simulink library "Pitch_TASK_Libs"  (Simulink 8.6)
settings: Solver=VariableStepAuto  SolverMode=SingleTasking  StartTime=0.0  StopTime=10.0  RelTol=1e-3
undefined symbols (not defined in the file or in its folder): M_SM_AUTO_RESET_TIME, M_SM_COUNTER_RESET_TIME
libraries: StandardLib x124, WindLib x7, Pitch_TASK_Libs x4, simulink x2
(part 1 of 2)
settings Model: Creator=300005582  LastModifiedBy=204050978

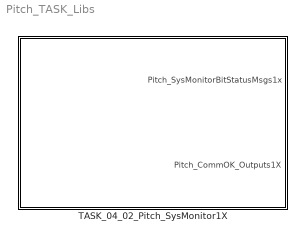
== system Pitch_TASK_Libs ==
  TASK_04_02_Pitch_SysMonitor1X : Subsystem  Priority=5
      settings: AttributesFormatString=ExecutionOrder = %<Priority>

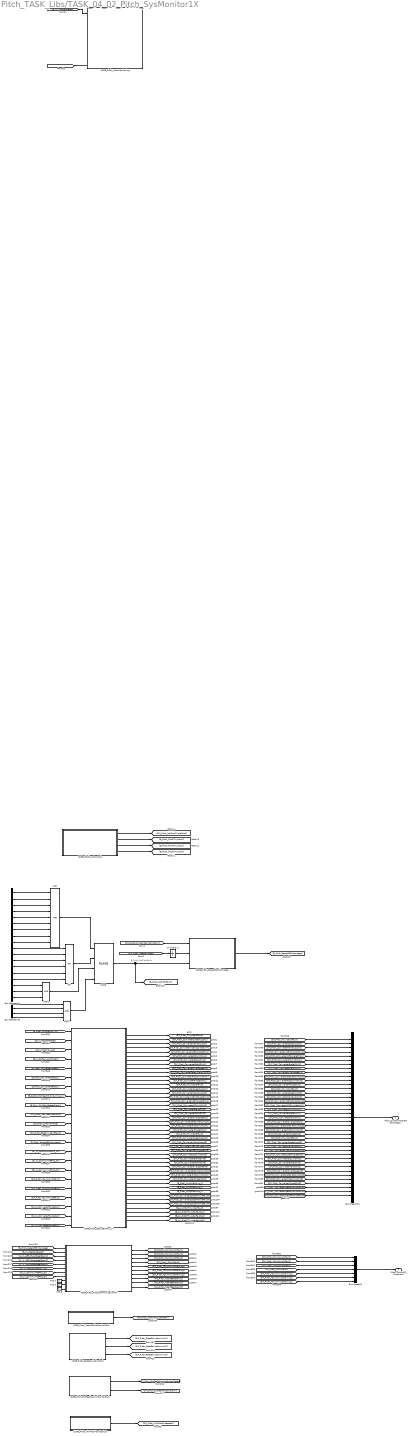
== system Pitch_TASK_Libs/TASK_04_02_Pitch_SysMonitor1X ==
  note: B_Pitch_NoPitchFault
  AND : StandardLib/Logical operations/AND  RepeatCnt=8  SampleTime=-1  ExecutionOrder=0
  AND1 : StandardLib/Logical operations/AND  RepeatCnt=3  SampleTime=-1  ExecutionOrder=0
  AND2 : StandardLib/Logical operations/AND  RepeatCnt=2  SampleTime=-1  ExecutionOrder=0
  Bus Creator10 : BusCreator  Inputs=39
  Bus Creator5 : BusCreator  Inputs=7  OutDataTypeStr=Bus: Pitch_CommOK_Outputs1X
  Bus Selector44 : BusSelector  OutputSignals=ExtInputs.DI_In_A1BattChargeOK,ExtInputs.DI_In_A2BattChargeOK,ExtInputs.DI_In_A3BattChargeOK,ExtInputs.DI_In_BattStringOKA1,ExtInputs.DI_In_BattStringOKA2,ExtInputs.DI_In_BattStringOKA3,ExtInputs.DI_In_BattVoltCompareOKA1,ExtInputs.DI_In_BattVoltCompareOKA2,ExtInputs.DI_In_BattVoltCompareOKA3,ExtInputs.DI_In_ConverterFaultedA1,ExtInputs.DI_In_ConverterFaultedA2,ExtInputs.DI_In_ConverterFaultedA3,ExtInputs.DI_In_MotorRTDFaultA1,ExtInputs.DI_In_MotorRTDFaultA2,ExtInputs.DI_In_MotorRTDFaultA3,ExtInputs.DI_In_CommunAEPA1_Ok,ExtInputs.DI_In_CommunAEPA2_Ok,ExtInputs.DI_In_CommunAEPA3_Ok
  Bus Selector45 : BusSelector  OutputSignals=Pitch_GlobalData.B_Pitch_Converter1Ready,Pitch_GlobalData.B_Pitch_Converter2Ready,Pitch_GlobalData.B_Pitch_Converter3Ready,OpCtl_GlobalData.B_OpCtl_PitchRectifyOnSummary
  OR : StandardLib/Logical operations/OR  RepeatCnt=5  SampleTime=-1  ExecutionOrder=0
  P13.1 : Constant  Value=0  OutDataTypeStr=boolean  SampleTime=-1
  P13.2 : Constant  Value=0  OutDataTypeStr=boolean  SampleTime=-1
  P13.3 : Constant  Value=0  OutDataTypeStr=boolean  SampleTime=-1
  RUNG : StandardLib/Logical operations/RUNG  Equation=A*(~B)*C*D  RepeatCount=4  SampleTime=-1  ExecutionOrder=0
  USRB_PitchSysMonStub : Subsystem  TreatAsAtomicUnit=on
      settings: MinAlgLoopOccurrences=on
  USRB_Pitch_ExtFeatherLimitSwitchStub : Subsystem  TreatAsAtomicUnit=on
  USRB_Pitch_MinPitchMonitorStub : Subsystem  TreatAsAtomicUnit=on
  USRB_Pitch_MotorCableMonitorStub : Subsystem  TreatAsAtomicUnit=on
  USRB_Pitch_MotorMonitoring : Subsystem  TreatAsAtomicUnit=on
  USRB_Pitch_PitchCommunicationOK : Subsystem  TreatAsAtomicUnit=on
  USRB_Pitch_RateDeviationStub : Subsystem  TreatAsAtomicUnit=on
  USRB_Pitch_ResetAftGridOutage : Subsystem  TreatAsAtomicUnit=on
  USRB_Pitch_StatusBitMon_1X : Subsystem  TreatAsAtomicUnit=on
  Unit Delay1 : UnitDelay  SampleTime=-1
  Pitch_SysMonitorBitStatusMsgs1x : Outport  OutDataTypeStr=Bus: Pitch_SysMonitor_LocalData1X
  Pitch_CommOK_Outputs1X : Outport  Port=2  OutDataTypeStr=Bus: Pitch_CommOK_Outputs1X
  wires:
  USRB_PitchSysMonStub/4(B_Pitch_PitchThysitor3) -> [B_Pitch_PitchThysitor3]  "B_Pitch_PitchThysitor3"
  USRB_PitchSysMonStub/2(B_Pitch_PitchThysitor1) -> [B_Pitch_PitchThysitor1]  "B_Pitch_PitchThysitor1"
  USRB_PitchSysMonStub/3(B_Pitch_PitchThysitor2) -> [B_Pitch_PitchThysitor2]  "B_Pitch_PitchThysitor2"
  USRB_PitchSysMonStub/1(SM_Pitch_MalfuncTriplePitch) -> [SM_Pitch_MalfuncTriplePitch]  "SM_Pitch_MalfuncTriplePitch"
  OR/1 -> RUNG/2
  AND/1 -> RUNG/1
  [SM_OpCtl_SystemReinitalization] -> USRB_Pitch_ResetAftGridOutage/1(SM_OpCtl_SystemReinitalization)
  USRB_Pitch_ResetAftGridOutage/1(B_Pitch_ResetAftGridoutage) -> [B_Pitch_ResetAftGridoutage]  "B_Pitch_ResetAftGridouate"
  Bus Selector44/1 -> AND/1  "<DI_In_A1BattChargeOK>"
  Bus Selector44/2 -> AND/2  "<DI_In_A2BattChargeOK>"
  Bus Selector44/3 -> AND/3  "<DI_In_A3BattChargeOK>"
  Bus Selector44/4 -> AND/4  "<DI_In_BattStringOKA1>"
  Bus Selector44/5 -> AND/5  "<DI_In_BattStringOKA2>"
  Bus Selector44/6 -> AND/6  "<DI_In_BattStringOKA3>"
  Bus Selector44/7 -> AND/7  "<DI_In_BattVoltCompareOKA1>"
  Bus Selector44/8 -> AND/8  "<DI_In_BattVoltCompareOKA2>"
  Bus Selector44/9 -> AND/9  "<DI_In_BattVoltCompareOKA3>"
  Bus Selector44/10 -> OR/1  "<DI_In_ConverterFaultedA1>"
  Bus Selector44/11 -> OR/2  "<DI_In_ConverterFaultedA2>"
  Bus Selector44/12 -> OR/3  "<DI_In_ConverterFaultedA3>"
  Bus Selector44/13 -> OR/4  "<DI_In_MotorRTDFaultA1>"
  Bus Selector44/14 -> OR/5  "<DI_In_MotorRTDFaultA2>"
  Bus Selector44/15 -> OR/6  "<DI_In_MotorRTDFaultA3>"
  RUNG/1 -> USRB_Pitch_ResetAftGridOutage/3(Pich_GeneralOK), [B_Pitch_NoPitchFault]
  Bus Selector45/1 -> AND1/1  "<B_Pitch_Converter1Ready>"
  Bus Selector45/2 -> AND1/2  "<B_Pitch_Converter2Ready>"
  Bus Selector45/3 -> AND1/3  "<B_Pitch_Converter3Ready>"
  Bus Selector45/4 -> AND1/4  "<B_OpCtl_PitchRectifyOnSummary>"
  Bus Selector44/16 -> AND2/1  "<DI_In_CommunAEPA1_Ok>"
  Bus Selector44/17 -> AND2/2  "<DI_In_CommunAEPA2_Ok>"
  Bus Selector44/18 -> AND2/3  "<DI_In_CommunAEPA3_Ok>"
  AND1/1 -> RUNG/4
  AND2/1 -> RUNG/3
  [SM_Pitch_InternalMode] -> Unit Delay1/1
  Unit Delay1/1 -> USRB_Pitch_ResetAftGridOutage/2(SM_Pitch_InternalMode)
  [B_Pitch_ResetAftGridoutage] -> ?
  [B_In_WtgStartReset] -> USRB_Pitch_MotorMonitoring/1(B_In_WtgStartReset)
  USRB_Pitch_StatusBitMon_1X/1(SM_Pitch_Thyristor1Fault) -> [SM_Pitch_Thyristor1Fault]  "SM_Pitch_Thyristor1Fault"
  USRB_Pitch_StatusBitMon_1X/2(SM_Pitch_ConverterSpeedLossA1) -> [SM_Pitch_ConverterSpeedLossA1]  "SM_Pitch_ConverterSpeedLossA1"
  USRB_Pitch_StatusBitMon_1X/3(SM_Pitch_ConverterMarkerLossA1) -> [SM_Pitch_ConverterMarkerLossA1]  "SM_Pitch_ConverterMarkerLossA1"
  USRB_Pitch_StatusBitMon_1X/4(SM_Pitch_ConverterIncEncCorrectionA1) -> [SM_Pitch_ConverterIncEncCorrectionA1]  "SM_Pitch_ConverterIncEncCorrectionA1"
  USRB_Pitch_StatusBitMon_1X/5(SM_Pitch_ConverterLS90AngleErrA1) -> [SM_Pitch_ConverterLS90AngleErrA1]  "SM_Pitch_ConverterLS90AngleErrA1"
  USRB_Pitch_StatusBitMon_1X/6(SM_Pitch_ConverterDCLinkOKA1) -> [SM_Pitch_ConverterDCLinkOKA1]  "SM_Pitch_ConverterDCLinkOKA1"
  USRB_Pitch_StatusBitMon_1X/7(SM_Pitch_ConverterBrakeOKA1) -> [SM_Pitch_ConverterBrakeOKA1]  "SM_Pitch_ConverterBrakeOKA1"
  USRB_Pitch_StatusBitMon_1X/8(SM_Pitch_ConverterFieldOKA1) -> [SM_Pitch_ConverterFieldOKA1]  "SM_Pitch_ConverterFieldOKA1"
  USRB_Pitch_StatusBitMon_1X/9(SM_Pitch_ConverterOverSpeedA1) -> [SM_Pitch_ConverterOverSpeedA1]  "SM_Pitch_ConverterOverSpeedA1"
  USRB_Pitch_StatusBitMon_1X/10(SM_Pitch_ConverterSafetyRelayPLCA1) -> [SM_Pitch_ConverterSafetyRelayPLCA1]  "SM_Pitch_ConverterSafetyRelayPLCA1"
  USRB_Pitch_StatusBitMon_1X/11(SM_Pitch_ConverterPICCommOKA1) -> [SM_Pitch_ConverterPICCommOKA1]  "SM_Pitch_ConverterPICCommOKA1"
  USRB_Pitch_StatusBitMon_1X/12(SM_Pitch_ConverterPhaseOkA1) -> [SM_Pitch_ConverterPhaseOkA1]  "SM_Pitch_ConverterPhaseOkA1"
  USRB_Pitch_StatusBitMon_1X/13(SM_Pitch_Thyristor2Fault) -> [SM_Pitch_Thyristor2Fault]  "SM_Pitch_Thyristor2Fault"
  USRB_Pitch_StatusBitMon_1X/14(SM_Pitch_ConverterSpeedLossA2) -> [SM_Pitch_ConverterSpeedLossA2]  "SM_Pitch_ConverterSpeedLossA2"
  USRB_Pitch_StatusBitMon_1X/15(SM_Pitch_ConverterMarkerLossA2) -> [SM_Pitch_ConverterMarkerLossA2]  "SM_Pitch_ConverterMarkerLossA2"
  USRB_Pitch_StatusBitMon_1X/16(SM_Pitch_ConverterIncEncCorrectionA2) -> [SM_Pitch_ConverterIncEncCorrectionA2]  "SM_Pitch_ConverterIncEncCorrectionA2"
  USRB_Pitch_StatusBitMon_1X/17(SM_Pitch_ConverterLS90AngleErrA2) -> [SM_Pitch_ConverterLS90AngleErrA2]  "SM_Pitch_ConverterLS90AngleErrA2"
  USRB_Pitch_StatusBitMon_1X/18(SM_Pitch_ConverterDCLinkOKA2) -> [SM_Pitch_ConverterDCLinkOKA2]  "SM_Pitch_ConverterDCLinkOKA2"
  USRB_Pitch_StatusBitMon_1X/19(SM_Pitch_ConverterBrakeOKA2) -> [SM_Pitch_ConverterBrakeOKA2]  "SM_Pitch_ConverterBrakeOKA2"
  USRB_Pitch_StatusBitMon_1X/20(SM_Pitch_ConverterFieldOKA2) -> [SM_Pitch_ConverterFieldOKA2]  "SM_Pitch_ConverterFieldOKA2"
  USRB_Pitch_StatusBitMon_1X/21(SM_Pitch_ConverterOverSpeedA2) -> [SM_Pitch_ConverterOverSpeedA2]  "SM_Pitch_ConverterOverSpeedA2"
  USRB_Pitch_StatusBitMon_1X/22(SM_Pitch_ConverterSafetyRelayPLCA2) -> [SM_Pitch_ConverterSafetyRelayPLCA2]  "SM_Pitch_ConverterSafetyRelayPLCA2"
  USRB_Pitch_StatusBitMon_1X/23(SM_Pitch_ConverterPICCommOKA2) -> [SM_Pitch_ConverterPICCommOKA2]  "SM_Pitch_ConverterPICCommOKA2"
  USRB_Pitch_StatusBitMon_1X/24(SM_Pitch_ConverterPhaseOkA2) -> [SM_Pitch_ConverterPhaseOkA2]  "SM_Pitch_ConverterPhaseOkA2"
  USRB_Pitch_StatusBitMon_1X/25(SM_Pitch_Thyristor3Fault) -> [SM_Pitch_Thyristor3Fault]  "SM_Pitch_Thyristor3Fault"
  USRB_Pitch_StatusBitMon_1X/26(SM_Pitch_ConverterSpeedLossA3) -> [SM_Pitch_ConverterSpeedLossA3]  "SM_Pitch_ConverterSpeedLossA3"
  USRB_Pitch_StatusBitMon_1X/27(SM_Pitch_ConverterMarkerLossA3) -> [SM_Pitch_ConverterMarkerLossA3]  "SM_Pitch_ConverterMarkerLossA3"
  USRB_Pitch_StatusBitMon_1X/28(SM_Pitch_ConverterIncEncCorrectionA3) -> [SM_Pitch_ConverterIncEncCorrectionA3]  "SM_Pitch_ConverterIncEncCorrectionA3"
  USRB_Pitch_StatusBitMon_1X/29(SM_Pitch_ConverterLS90AngleErrA3) -> [SM_Pitch_ConverterLS90AngleErrA3]  "SM_Pitch_ConverterLS90AngleErrA3"
  USRB_Pitch_StatusBitMon_1X/30(SM_Pitch_ConverterDCLinkOKA3) -> [SM_Pitch_ConverterDCLinkOKA3]  "SM_Pitch_ConverterDCLinkOKA3"
  USRB_Pitch_StatusBitMon_1X/31(SM_Pitch_ConverterBrakeOKA3) -> [SM_Pitch_ConverterBrakeOKA3]  "SM_Pitch_ConverterBrakeOKA3"
  USRB_Pitch_StatusBitMon_1X/32(SM_Pitch_ConverterFieldOKA3) -> [SM_Pitch_ConverterFieldOKA3]  "SM_Pitch_ConverterFieldOKA3"
  USRB_Pitch_StatusBitMon_1X/33(SM_Pitch_ConverterOverSpeedA3) -> [SM_Pitch_ConverterOverSpeedA3]  "SM_Pitch_ConverterOverSpeedA3"
  USRB_Pitch_StatusBitMon_1X/34(SM_Pitch_ConverterSafetyRelayPLCA3) -> [SM_Pitch_ConverterSafetyRelayPLCA3]  "SM_Pitch_ConverterSafetyRelayPLCA3"
  USRB_Pitch_StatusBitMon_1X/35(SM_Pitch_ConverterPICCommOKA3) -> [SM_Pitch_ConverterPICCommOKA3]  "SM_Pitch_ConverterPICCommOKA3"
  USRB_Pitch_StatusBitMon_1X/36(SM_Pitch_ConverterPhaseOkA3) -> [SM_Pitch_ConverterPhaseOkA3]  "SM_Pitch_ConverterPhaseOkA3"
  USRB_Pitch_StatusBitMon_1X/37(B_Pitch_Axis1Malfunc_L) -> [B_Pitch_Axis1Malfunc_L]
  USRB_Pitch_StatusBitMon_1X/38(B_Pitch_Axis2Malfunc_L) -> [B_Pitch_Axis2Malfunc_L]
  USRB_Pitch_StatusBitMon_1X/39(B_Pitch_Axis3Malfunc_L) -> [B_Pitch_Axis3Malfunc_L]
  [B_Pitch_AxisMalFun_LL] -> USRB_Pitch_StatusBitMon_1X/1(B_Pitch_AxisMalFun_LL)
  [B_In_WtgStartReset] -> USRB_Pitch_StatusBitMon_1X/2(B_In_WtgStartReset)
  [C_In_PitchManual] -> USRB_Pitch_StatusBitMon_1X/3(C_In_PitchManual)
  [B_In_SafetyLoopClosed] -> USRB_Pitch_StatusBitMon_1X/4(B_In_SafetyLoopClosed)
  [B_Pitch_Converter1Ready] -> USRB_Pitch_StatusBitMon_1X/5(B_Pitch_Converter1Ready)
  [B_Pitch_Converter2Ready] -> USRB_Pitch_StatusBitMon_1X/6(B_Pitch_Converter2Ready)
  [B_Pitch_Converter3Ready] -> USRB_Pitch_StatusBitMon_1X/7(B_Pitch_Converter3Ready)
  [B_OpCtl_PitchRectifyOnSummary] -> USRB_Pitch_StatusBitMon_1X/8(B_OpCtl_PitchRectifyOnSummary)
  [B_Envr_GridFaultResetDelay] -> USRB_Pitch_StatusBitMon_1X/9(B_Envr_GridFaultResetDelay)
  [SM_Pitch_ServiceSwitchHub] -> USRB_Pitch_StatusBitMon_1X/10(SM_Pitch_ServiceSwitchHub)
  [SM_Pitch_InternalMode] -> USRB_Pitch_StatusBitMon_1X/11(SM_Pitch_InternalMode)
  [SM_Pitch_BattDriveGridFault] -> USRB_Pitch_StatusBitMon_1X/12(SM_Pitch_BattDriveGridFault)
  [B_Pitch_ResetAftGridoutage] -> USRB_Pitch_StatusBitMon_1X/13(B_Pitch_ResetAftGridoutage)
  [DI_In_CommunAEPA1_Ok] -> USRB_Pitch_StatusBitMon_1X/14(DI_In_CommunAEPA1_Ok)
  [DI_In_CommunAEPA2_Ok] -> USRB_Pitch_StatusBitMon_1X/15(DI_In_CommunAEPA2_Ok)
  [DI_In_CommunAEPA3_Ok] -> USRB_Pitch_StatusBitMon_1X/16(DI_In_CommunAEPA3_Ok)
  [SM_Pitch_IOLinkAxis1Fault] -> USRB_Pitch_StatusBitMon_1X/17(SM_Pitch_IOLinkAxis1Fault)
  [SM_Pitch_IOLinkAxis2Fault] -> USRB_Pitch_StatusBitMon_1X/18(SM_Pitch_IOLinkAxis2Fault)
  [SM_Pitch_IOLinkAxis3Fault] -> USRB_Pitch_StatusBitMon_1X/19(SM_Pitch_IOLinkAxis3Fault)
  [DI_In_ConverterFaultedA1] -> USRB_Pitch_StatusBitMon_1X/20(DI_In_ConverterFaultedA1)
  [DI_In_ConverterFaultedA2] -> USRB_Pitch_StatusBitMon_1X/21(DI_In_ConverterFaultedA2)
  [DI_In_ConverterFaultedA3] -> USRB_Pitch_StatusBitMon_1X/22(DI_In_ConverterFaultedA3)
  USRB_Pitch_StatusBitMon_1X/43(B_AnyPitchThyristorFault) -> [B_AnyPitchThyristorFault]
  USRB_Pitch_PitchCommunicationOK/1(SM_Pitch_IOLinkAxis1Fault) -> [SM_Pitch_IOLinkAxis1Fault]
  USRB_Pitch_PitchCommunicationOK/2(SM_Pitch_IOLinkAxis2Fault) -> [SM_Pitch_IOLinkAxis2Fault]
  USRB_Pitch_PitchCommunicationOK/3(SM_Pitch_IOLinkAxis3Fault) -> [SM_Pitch_IOLinkAxis3Fault]
  USRB_Pitch_PitchCommunicationOK/4(SM_Pitch_IOLinkFault) -> [SM_Pitch_IOLinkFault]
  USRB_Pitch_PitchCommunicationOK/5(SM_Pitch_IOLinkAxis1Warning) -> [SM_Pitch_IOLinkAxis1Warning]
  USRB_Pitch_PitchCommunicationOK/6(SM_Pitch_IOLinkAxis2Warning) -> [SM_Pitch_IOLinkAxis2Warning]
  USRB_Pitch_PitchCommunicationOK/7(SM_Pitch_IOLinkAxis3Warning) -> [SM_Pitch_IOLinkAxis3Warning]
  USRB_Pitch_PitchCommunicationOK/8(AO_Pitch_HeartBeatSend1) -> [AO_Pitch_HeartBeatSend1]
  USRB_Pitch_PitchCommunicationOK/9(AO_Pitch_HeartBeatSend2) -> [AO_Pitch_HeartBeatSend2]
  USRB_Pitch_PitchCommunicationOK/10(AO_Pitch_HeartBeatSend3) -> [AO_Pitch_HeartBeatSend3]
  [B_Pitch_ResetAftGridoutage] -> USRB_Pitch_PitchCommunicationOK/1(B_Pitch_ResetAftGridoutage)
  [B_In_WtgStartReset] -> USRB_Pitch_PitchCommunicationOK/2(B_In_WtgStartReset)
  [AI_In_AEPAHeartbeatRecv1] -> USRB_Pitch_PitchCommunicationOK/3(AI_In_AEPAHeartbeatRecv1)
  [AI_In_AEPAHeartbeatRecv2] -> USRB_Pitch_PitchCommunicationOK/4(AI_In_AEPAHeartbeatRecv2)
  [AI_In_AEPAHeartbeatRecv3] -> USRB_Pitch_PitchCommunicationOK/5(AI_In_AEPAHeartbeatRecv3)
  [DI_In_CommunAEPA1_Ok] -> USRB_Pitch_PitchCommunicationOK/6(DI_In_CommunAEPA1_Ok)
  [DI_In_CommunAEPA2_Ok] -> USRB_Pitch_PitchCommunicationOK/7(DI_In_CommunAEPA2_Ok)
  [DI_In_CommunAEPA3_Ok] -> USRB_Pitch_PitchCommunicationOK/8(DI_In_CommunAEPA3_Ok)
  P13.1/1 -> USRB_Pitch_PitchCommunicationOK/9(B_TestShortTimeComFault)
  P13.2/1 -> USRB_Pitch_PitchCommunicationOK/10(B_TestLongTimeComFaultTwoAxes)
  P13.3/1 -> USRB_Pitch_PitchCommunicationOK/11(B_TestLongTimeComFaultAllAxes)
  Bus Creator10/1 -> Pitch_SysMonitorBitStatusMsgs1x/1  "Pitch_SysMonitorBitStatusMsgs1x"
  [SM_Pitch_Thyristor1Fault] -> Bus Creator10/1  "SM_Pitch_Thyristor1Fault"
  [SM_Pitch_ConverterSpeedLossA1] -> Bus Creator10/2  "SM_Pitch_ConverterSpeedLossA1"
  [SM_Pitch_ConverterMarkerLossA1] -> Bus Creator10/3  "SM_Pitch_ConverterMarkerLossA1"
  [SM_Pitch_ConverterIncEncCorrectionA1] -> Bus Creator10/4  "SM_Pitch_ConverterIncEncCorrectionA1"
  [SM_Pitch_ConverterLS90AngleErrA1] -> Bus Creator10/5  "SM_Pitch_ConverterLS90AngleErrA1"
  [SM_Pitch_ConverterDCLinkOKA1] -> Bus Creator10/6  "SM_Pitch_ConverterDCLinkOKA1"
  [SM_Pitch_ConverterBrakeOKA1] -> Bus Creator10/7  "SM_Pitch_ConverterBrakeOKA1"
  [SM_Pitch_ConverterFieldOKA1] -> Bus Creator10/8  "SM_Pitch_ConverterFieldOKA1"
  [SM_Pitch_ConverterOverSpeedA1] -> Bus Creator10/9  "SM_Pitch_ConverterOverSpeedA1"
  [SM_Pitch_ConverterSafetyRelayPLCA1] -> Bus Creator10/10  "SM_Pitch_ConverterSafetyRelayPLCA1"
  [SM_Pitch_ConverterPICCommOKA1] -> Bus Creator10/11  "SM_Pitch_ConverterPICCommOKA1"
  [SM_Pitch_ConverterPhaseOkA1] -> Bus Creator10/12  "SM_Pitch_ConverterPhaseOkA1"
  [SM_Pitch_Thyristor2Fault] -> Bus Creator10/13  "SM_Pitch_Thyristor2Fault"
  [SM_Pitch_ConverterSpeedLossA2] -> Bus Creator10/14  "SM_Pitch_ConverterSpeedLossA2"
  [SM_Pitch_ConverterMarkerLossA2] -> Bus Creator10/15  "SM_Pitch_ConverterMarkerLossA2"
  [SM_Pitch_ConverterIncEncCorrectionA2] -> Bus Creator10/16  "SM_Pitch_ConverterIncEncCorrectionA2"
  [SM_Pitch_ConverterLS90AngleErrA2] -> Bus Creator10/17  "SM_Pitch_ConverterLS90AngleErrA2"
  [SM_Pitch_ConverterDCLinkOKA2] -> Bus Creator10/18  "SM_Pitch_ConverterDCLinkOKA2"
  [SM_Pitch_ConverterBrakeOKA2] -> Bus Creator10/19  "SM_Pitch_ConverterBrakeOKA2"
  [SM_Pitch_ConverterFieldOKA2] -> Bus Creator10/20  "SM_Pitch_ConverterFieldOKA2"
  [SM_Pitch_ConverterOverSpeedA2] -> Bus Creator10/21  "SM_Pitch_ConverterOverSpeedA2"
  [SM_Pitch_ConverterSafetyRelayPLCA2] -> Bus Creator10/22  "SM_Pitch_ConverterSafetyRelayPLCA2"
  [SM_Pitch_ConverterPICCommOKA2] -> Bus Creator10/23  "SM_Pitch_ConverterPICCommOKA2"
  [SM_Pitch_ConverterPhaseOkA2] -> Bus Creator10/24  "SM_Pitch_ConverterPhaseOkA2"
  [SM_Pitch_Thyristor3Fault] -> Bus Creator10/25  "SM_Pitch_Thyristor3Fault"
  [SM_Pitch_ConverterSpeedLossA3] -> Bus Creator10/26  "SM_Pitch_ConverterSpeedLossA3"
  [SM_Pitch_ConverterMarkerLossA3] -> Bus Creator10/27  "SM_Pitch_ConverterMarkerLossA3"
  [SM_Pitch_ConverterIncEncCorrectionA3] -> Bus Creator10/28  "SM_Pitch_ConverterIncEncCorrectionA3"
  [SM_Pitch_ConverterLS90AngleErrA3] -> Bus Creator10/29  "SM_Pitch_ConverterLS90AngleErrA3"
  [SM_Pitch_ConverterDCLinkOKA3] -> Bus Creator10/30  "SM_Pitch_ConverterDCLinkOKA3"
  [SM_Pitch_ConverterBrakeOKA3] -> Bus Creator10/31  "SM_Pitch_ConverterBrakeOKA3"
  [SM_Pitch_ConverterFieldOKA3] -> Bus Creator10/32  "SM_Pitch_ConverterFieldOKA3"
  [SM_Pitch_ConverterOverSpeedA3] -> Bus Creator10/33  "SM_Pitch_ConverterOverSpeedA3"
  [SM_Pitch_ConverterSafetyRelayPLCA3] -> Bus Creator10/34  "SM_Pitch_ConverterSafetyRelayPLCA3"
  [SM_Pitch_ConverterPICCommOKA3] -> Bus Creator10/35  "SM_Pitch_ConverterPICCommOKA3"
  [SM_Pitch_ConverterPhaseOkA3] -> Bus Creator10/36  "SM_Pitch_ConverterPhaseOkA3"
  USRB_Pitch_StatusBitMon_1X/40(SM_Pitch_ConverterSpeedProfileFaultA1) -> [SM_Pitch_ConverterSpeedProfileFaultA1]
  USRB_Pitch_StatusBitMon_1X/41(SM_Pitch_ConverterSpeedProfileFaultA2) -> [SM_Pitch_ConverterSpeedProfileFaultA2]
  USRB_Pitch_StatusBitMon_1X/42(SM_Pitch_ConverterSpeedProfileFaultA3) -> [SM_Pitch_ConverterSpeedProfileFaultA3]
  [SM_Pitch_ConverterSpeedProfileFaultA1] -> Bus Creator10/37  "SM_Pitch_ConverterSpeedProfileFaultA1"
  [SM_Pitch_ConverterSpeedProfileFaultA2] -> Bus Creator10/38  "SM_Pitch_ConverterSpeedProfileFaultA2"
  [SM_Pitch_ConverterSpeedProfileFaultA3] -> Bus Creator10/39  "SM_Pitch_ConverterSpeedProfileFaultA3"
  USRB_Pitch_StatusBitMon_1X/44(B_AnyPitchThyristorFaultA1) -> [B_AnyPitchThyristorFaultA1]
  USRB_Pitch_StatusBitMon_1X/45(B_AnyPitchThyristorFaultA2) -> [B_AnyPitchThyristorFaultA2]
  USRB_Pitch_StatusBitMon_1X/46(B_AnyPitchThyristorFaultA3) -> [B_AnyPitchThyristorFaultA3]
  USRB_Pitch_MotorCableMonitorStub/1(SM_Pitch_PitchMotorCableFail) -> [SM_Pitch_PitchMotorCableFail]
  USRB_Pitch_RateDeviationStub/1(SM_Pitch_RateDeviationAxis1) -> [SM_Pitch_RateDeviationAxis1]
  USRB_Pitch_RateDeviationStub/2(SM_Pitch_RateDeviationAxis2) -> [SM_Pitch_RateDeviationAxis2]
  USRB_Pitch_RateDeviationStub/3(SM_Pitch_RateDeviationAxis3) -> [SM_Pitch_RateDeviationAxis3]
  USRB_Pitch_ExtFeatherLimitSwitchStub/1(SM_Pitch_ExtFeathPosLmtSwitchDefect) -> [SM_Pitch_ExtFeathPosLmtSwitchDefect]
  USRB_Pitch_ExtFeatherLimitSwitchStub/2(SM_Pitch_ExtFeathPosOverRun) -> [SM_Pitch_ExtFeathPosOverRun]
  USRB_Pitch_MinPitchMonitorStub/1(SM_Pitch_MinPitchExceeded) -> [SM_Pitch_MinPitchExceeded]
  [SM_Pitch_IOLinkAxis1Fault] -> Bus Creator5/1  "SM_Pitch_IOLinkAxis1Fault"
  [SM_Pitch_IOLinkAxis2Fault] -> Bus Creator5/2  "SM_Pitch_IOLinkAxis2Fault"
  [SM_Pitch_IOLinkAxis3Fault] -> Bus Creator5/3  "SM_Pitch_IOLinkAxis3Fault"
  [SM_Pitch_IOLinkFault] -> Bus Creator5/4  "SM_Pitch_IOLinkFault"
  [SM_Pitch_IOLinkAxis1Warning] -> Bus Creator5/5  "SM_Pitch_IOLinkAxis1Warning"
  [SM_Pitch_IOLinkAxis2Warning] -> Bus Creator5/6  "SM_Pitch_IOLinkAxis2Warning"
  [SM_Pitch_IOLinkAxis3Warning] -> Bus Creator5/7  "SM_Pitch_IOLinkAxis3Warning"
  Bus Creator5/1 -> Pitch_CommOK_Outputs1X/1  "Pitch_CommOK_Outputs1X"

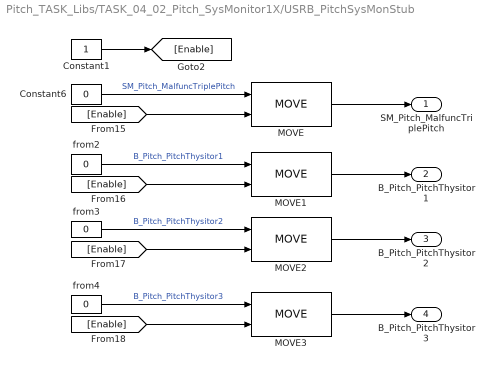
== system Pitch_TASK_Libs/TASK_04_02_Pitch_SysMonitor1X/USRB_PitchSysMonStub ==
  Constant1 : Constant  OutDataTypeStr=boolean
  Constant6 : Constant  Value=0  OutDataTypeStr=boolean
  MOVE{,1..3} (4 alike) : StandardLib/Memory operations/MOVE  DataType=BOOLEAN  SampleTime=-1  ExecutionOrder=0
  from2 : Constant  Value=0  OutDataTypeStr=boolean
  from3 : Constant  Value=0  OutDataTypeStr=boolean
  from4 : Constant  Value=0  OutDataTypeStr=boolean
  SM_Pitch_MalfuncTriplePitch : Outport  OutDataTypeStr=boolean
  B_Pitch_PitchThysitor1 : Outport  Port=2  OutDataTypeStr=boolean
  B_Pitch_PitchThysitor2 : Outport  Port=3  OutDataTypeStr=boolean
  B_Pitch_PitchThysitor3 : Outport  Port=4  OutDataTypeStr=boolean
  wires:
  from2/1 -> MOVE1/1  "B_Pitch_PitchThysitor1"
  from3/1 -> MOVE2/1  "B_Pitch_PitchThysitor2"
  from4/1 -> MOVE3/1  "B_Pitch_PitchThysitor3"
  Constant6/1 -> MOVE/1  "SM_Pitch_MalfuncTriplePitch"
  [Enable] -> MOVE/2
  [Enable] -> MOVE1/2
  [Enable] -> MOVE2/2
  [Enable] -> MOVE3/2
  MOVE/1 -> SM_Pitch_MalfuncTriplePitch/1
  MOVE1/1 -> B_Pitch_PitchThysitor1/1
  MOVE2/1 -> B_Pitch_PitchThysitor2/1
  MOVE3/1 -> B_Pitch_PitchThysitor3/1
  Constant1/1 -> [Enable]

== system Pitch_TASK_Libs/TASK_04_02_Pitch_SysMonitor1X/USRB_Pitch_ExtFeatherLimitSwitchStub ==
  Constant1 : Constant  Value=0  OutDataTypeStr=boolean
  Constant18 : Constant  Value=0  OutDataTypeStr=boolean
  Constant19 : Constant  OutDataTypeStr=boolean
  Constant2 : Constant  OutDataTypeStr=boolean
  MOVE1 : StandardLib/Memory operations/MOVE  DataType=BOOLEAN  SampleTime=-1  ExecutionOrder=0
  MOVE9 : StandardLib/Memory operations/MOVE  DataType=BOOLEAN  SampleTime=-1  ExecutionOrder=0
  SM_Pitch_ExtFeathPosLmtSwitchDefect : Outport  OutDataTypeStr=boolean
  SM_Pitch_ExtFeathPosOverRun : Outport  Port=2  OutDataTypeStr=boolean
  wires:
  Constant19/1 -> MOVE9/2
  Constant18/1 -> MOVE9/1
  MOVE9/1 -> SM_Pitch_ExtFeathPosLmtSwitchDefect/1
  Constant2/1 -> MOVE1/2
  Constant1/1 -> MOVE1/1
  MOVE1/1 -> SM_Pitch_ExtFeathPosOverRun/1

== system Pitch_TASK_Libs/TASK_04_02_Pitch_SysMonitor1X/USRB_Pitch_MinPitchMonitorStub ==
  note: ***********************************************************************************************************************************************
      | ***********         Change history. Please include your changes below and in the in the modified Task / USRB         ***********
      | ***********************************************************************************************************************************************
      | 2013-01-11, JGC: Corrected logic of SM450. SUB block substituted by ADD block in threshold calculation
      | 2013-07-25, JGC: SM450 is masked during 5s after LVRT
  Constant18 : Constant  Value=0  OutDataTypeStr=boolean
  Constant19 : Constant  OutDataTypeStr=boolean
  MOVE9 : StandardLib/Memory operations/MOVE  DataType=BOOLEAN  SampleTime=-1  ExecutionOrder=0
  SM_Pitch_MinPitchExceeded : Outport  OutDataTypeStr=boolean
  wires:
  Constant19/1 -> MOVE9/2
  Constant18/1 -> MOVE9/1
  MOVE9/1 -> SM_Pitch_MinPitchExceeded/1

== system Pitch_TASK_Libs/TASK_04_02_Pitch_SysMonitor1X/USRB_Pitch_MotorCableMonitorStub ==
  Constant18 : Constant  Value=0  OutDataTypeStr=boolean
  Constant19 : Constant  OutDataTypeStr=boolean
  MOVE9 : StandardLib/Memory operations/MOVE  DataType=BOOLEAN  SampleTime=-1  ExecutionOrder=0
  SM_Pitch_PitchMotorCableFail : Outport  OutDataTypeStr=boolean
  wires:
  Constant19/1 -> MOVE9/2
  Constant18/1 -> MOVE9/1
  MOVE9/1 -> SM_Pitch_PitchMotorCableFail/1

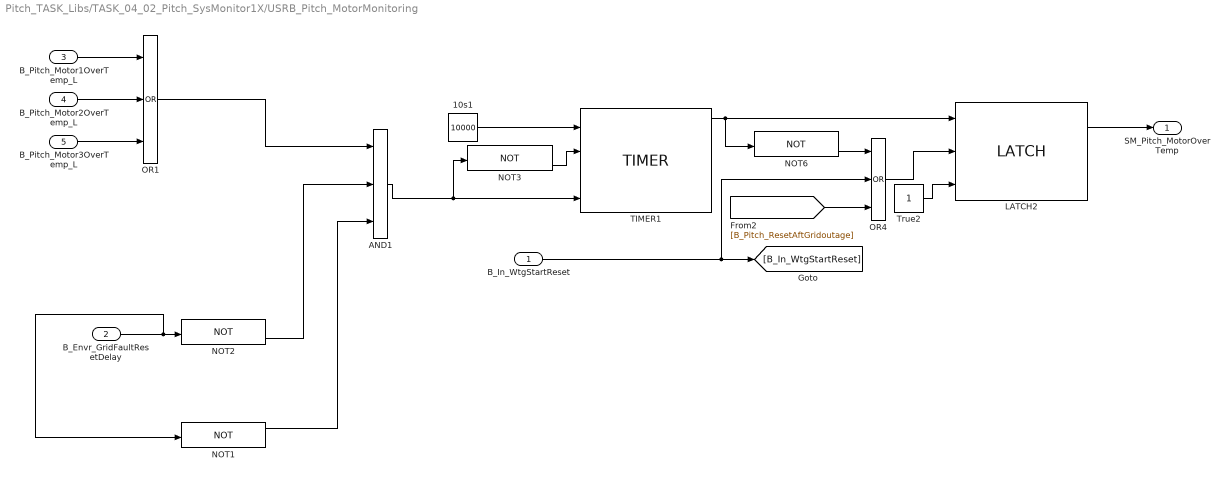
== system Pitch_TASK_Libs/TASK_04_02_Pitch_SysMonitor1X/USRB_Pitch_MotorMonitoring ==
  B_In_WtgStartReset : Inport  OutDataTypeStr=boolean
  B_Envr_GridFaultResetDelay : Inport  Port=2  OutDataTypeStr=boolean
  B_Pitch_Motor1OverTemp_L : Inport  Port=3  OutDataTypeStr=boolean
  B_Pitch_Motor2OverTemp_L : Inport  Port=4  OutDataTypeStr=boolean
  B_Pitch_Motor3OverTemp_L : Inport  Port=5  OutDataTypeStr=boolean
  10s1 : Constant  Value=10000  OutDataTypeStr=uint32  SampleTime=-1
  AND1 : StandardLib/Logical operations/AND  RepeatCnt=2  SampleTime=-1  ExecutionOrder=0
  LATCH2 : StandardLib/Logical operations/LATCH  SampleTime=-1  ExecutionOrder=0
  NOT{1..3,6} (4 alike) : StandardLib/Logical operations/NOT  SampleTime=-1  ExecutionOrder=0
  OR1 : StandardLib/Logical operations/OR  RepeatCnt=2  SampleTime=-1  ExecutionOrder=0
  OR4 : StandardLib/Logical operations/OR  RepeatCnt=2  SampleTime=-1  ExecutionOrder=0
  TIMER1 : StandardLib/Timers and Counters/TIMER  SampleTime=-1  ExecutionOrder=0
  True2 : Constant  OutDataTypeStr=boolean  SampleTime=-1
  SM_Pitch_MotorOverTemp : Outport  OutDataTypeStr=boolean
  wires:
  NOT6/2 -> OR4/1
  TIMER1/1 -> LATCH2/1, NOT6/1
  B_In_WtgStartReset/1 -> [B_In_WtgStartReset], OR4/2
  B_Pitch_Motor3OverTemp_L/1 -> OR1/3
  B_Pitch_Motor2OverTemp_L/1 -> OR1/2
  B_Pitch_Motor1OverTemp_L/1 -> OR1/1
  NOT3/2 -> TIMER1/2
  10s1/1 -> TIMER1/1
  AND1/1 -> NOT3/1, TIMER1/4
  B_Envr_GridFaultResetDelay/1 -> NOT1/1, NOT2/1
  LATCH2/1 -> SM_Pitch_MotorOverTemp/1
  True2/1 -> LATCH2/3
  NOT2/2 -> AND1/2
  OR1/1 -> AND1/1
  [B_Pitch_ResetAftGridoutage] -> OR4/3
  OR4/1 -> LATCH2/2
  NOT1/1 -> AND1/3

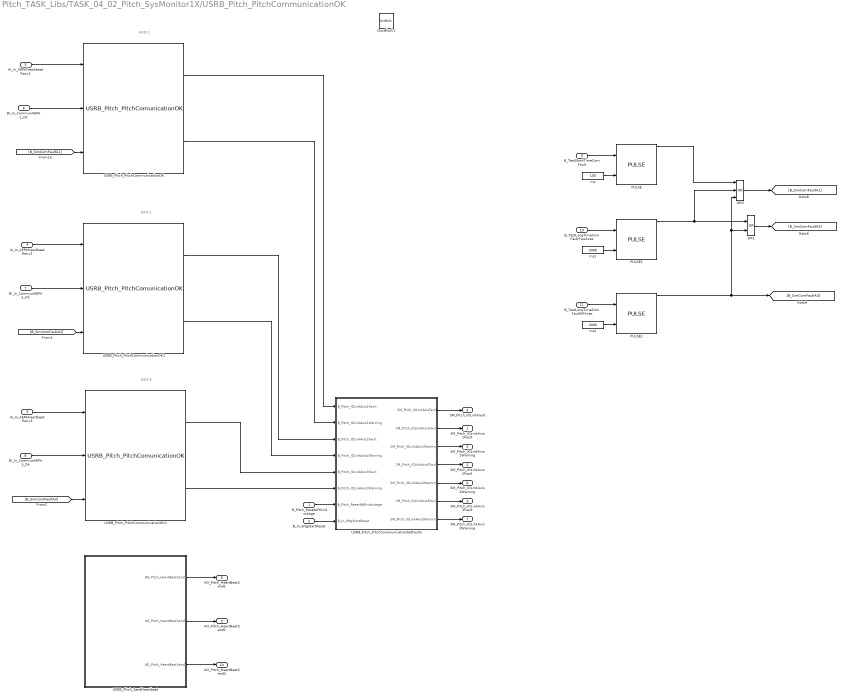
== system Pitch_TASK_Libs/TASK_04_02_Pitch_SysMonitor1X/USRB_Pitch_PitchCommunicationOK ==
  note: AXIS 1
  note: AXIS 2
  note: AXIS 3
  B_Pitch_ResetAftGridoutage : Inport  OutDataTypeStr=boolean
  B_In_WtgStartReset : Inport  Port=2  OutDataTypeStr=boolean
  AI_In_AEPAHeartbeatRecv1 : Inport  Port=3  OutDataTypeStr=int32
  AI_In_AEPAHeartbeatRecv2 : Inport  Port=4  OutDataTypeStr=int32
  AI_In_AEPAHeartbeatRecv3 : Inport  Port=5  OutDataTypeStr=int32
  DI_In_CommunAEPA1_Ok : Inport  Port=6  OutDataTypeStr=boolean
  DI_In_CommunAEPA2_Ok : Inport  Port=7  OutDataTypeStr=boolean
  DI_In_CommunAEPA3_Ok : Inport  Port=8  OutDataTypeStr=boolean
  B_TestShortTimeComFault : Inport  Port=9  OutDataTypeStr=boolean
  B_TestLongTimeComFaultTwoAxes : Inport  Port=10  OutDataTypeStr=boolean
  B_TestLongTimeComFaultAllAxes : Inport  Port=11  OutDataTypeStr=boolean
  DocBlock1 : simulink/Model-Wide Utilities/DocBlock  SystemSampleTime=-1  DocumentType=Text
  OR1 : StandardLib/Logical operations/OR  RepeatCnt=1  SampleTime=-1  ExecutionOrder=0
  OR3 : StandardLib/Logical operations/OR  RepeatCnt=2  SampleTime=-1  ExecutionOrder=0
  PULSE : StandardLib/Sequencing/PULSE  SampleTime=-1  ExecutionOrder=0
  PULSE1 : StandardLib/Sequencing/PULSE  SampleTime=-1  ExecutionOrder=0
  PULSE2 : StandardLib/Sequencing/PULSE  SampleTime=-1  ExecutionOrder=0
  USRB_Pitch_PitchCommunicationOK : WindLib/USRB_Pitch_PitchComunicationOK  SystemSampleTime=-1
  USRB_Pitch_PitchCommunicationOK1 : WindLib/USRB_Pitch_PitchComunicationOK  SystemSampleTime=-1
  USRB_Pitch_PitchCommunicationOK2 : WindLib/USRB_Pitch_PitchComunicationOK  SystemSampleTime=-1
  USRB_Pitch_PitchCommunicationSetFaults : Subsystem  TreatAsAtomicUnit=on
  USRB_Pitch_SendHeartbeat : Subsystem  TreatAsAtomicUnit=on
  ms : Constant  Value=130  OutDataTypeStr=uint32  SampleTime=-1
  ms1 : Constant  Value=2000  OutDataTypeStr=uint32  SampleTime=-1
  ms2 : Constant  Value=2000  OutDataTypeStr=uint32  SampleTime=-1
  SM_Pitch_IOLinkAxis1Fault : Outport  OutDataTypeStr=boolean
  SM_Pitch_IOLinkAxis2Fault : Outport  Port=2  OutDataTypeStr=boolean
  SM_Pitch_IOLinkAxis3Fault : Outport  Port=3  OutDataTypeStr=boolean
  SM_Pitch_IOLinkFault : Outport  Port=4  OutDataTypeStr=boolean
  SM_Pitch_IOLinkAxis1Warning : Outport  Port=5  OutDataTypeStr=boolean
  SM_Pitch_IOLinkAxis2Warning : Outport  Port=6  OutDataTypeStr=boolean
  SM_Pitch_IOLinkAxis3Warning : Outport  Port=7  OutDataTypeStr=boolean
  AO_Pitch_HeartBeatSend1 : Outport  Port=8  OutDataTypeStr=int32
  AO_Pitch_HeartBeatSend2 : Outport  Port=9  OutDataTypeStr=int32
  AO_Pitch_HeartBeatSend3 : Outport  Port=10  OutDataTypeStr=int32
  wires:
  [B_SimComFaultA3] -> USRB_Pitch_PitchCommunicationOK2/3
  DI_In_CommunAEPA3_Ok/1 -> USRB_Pitch_PitchCommunicationOK2/2
  [B_SimComFaultA2] -> USRB_Pitch_PitchCommunicationOK1/3
  DI_In_CommunAEPA2_Ok/1 -> USRB_Pitch_PitchCommunicationOK1/2
  [B_SimComFaultA1] -> USRB_Pitch_PitchCommunicationOK/3
  DI_In_CommunAEPA1_Ok/1 -> USRB_Pitch_PitchCommunicationOK/2
  USRB_Pitch_PitchCommunicationSetFaults/7(SM_Pitch_IOLinkAxis3Warning) -> SM_Pitch_IOLinkAxis3Warning/1
  USRB_Pitch_PitchCommunicationSetFaults/6(SM_Pitch_IOLinkAxis3Fault) -> SM_Pitch_IOLinkAxis3Fault/1
  USRB_Pitch_PitchCommunicationSetFaults/5(SM_Pitch_IOLinkAxis2Warning) -> SM_Pitch_IOLinkAxis2Warning/1
  USRB_Pitch_PitchCommunicationSetFaults/4(SM_Pitch_IOLinkAxis2Fault) -> SM_Pitch_IOLinkAxis2Fault/1
  USRB_Pitch_PitchCommunicationSetFaults/3(SM_Pitch_IOLinkAxis1Warning) -> SM_Pitch_IOLinkAxis1Warning/1
  USRB_Pitch_PitchCommunicationSetFaults/2(SM_Pitch_IOLinkAxis1Fault) -> SM_Pitch_IOLinkAxis1Fault/1
  USRB_Pitch_PitchCommunicationSetFaults/1(SM_Pitch_IOLinkAxisFault) -> SM_Pitch_IOLinkFault/1
  USRB_Pitch_PitchCommunicationOK2/2 -> USRB_Pitch_PitchCommunicationSetFaults/6(B_Pitch_IOLinkAxis3Warning)
  USRB_Pitch_SendHeartbeat/3(AO_Pitch_HeartBeatSend3) -> AO_Pitch_HeartBeatSend3/1
  USRB_Pitch_SendHeartbeat/2(AO_Pitch_HeartBeatSend2) -> AO_Pitch_HeartBeatSend2/1
  USRB_Pitch_SendHeartbeat/1(AO_Pitch_HeartBeatSend1) -> AO_Pitch_HeartBeatSend1/1
  B_In_WtgStartReset/1 -> USRB_Pitch_PitchCommunicationSetFaults/8(B_In_WtgStartReset)
  B_Pitch_ResetAftGridoutage/1 -> USRB_Pitch_PitchCommunicationSetFaults/7(B_Pitch_ResetAftGridoutage)
  USRB_Pitch_PitchCommunicationOK2/1 -> USRB_Pitch_PitchCommunicationSetFaults/5(B_Pitch_IOLinkAxis3Fault)
  USRB_Pitch_PitchCommunicationOK1/2 -> USRB_Pitch_PitchCommunicationSetFaults/4(B_Pitch_IOLinkAxis2Warning)
  USRB_Pitch_PitchCommunicationOK1/1 -> USRB_Pitch_PitchCommunicationSetFaults/3(B_Pitch_IOLinkAxis2Fault)
  USRB_Pitch_PitchCommunicationOK/2 -> USRB_Pitch_PitchCommunicationSetFaults/2(B_Pitch_IOLinkAxis1Warning)
  USRB_Pitch_PitchCommunicationOK/1 -> USRB_Pitch_PitchCommunicationSetFaults/1(B_Pitch_IOLinkAxis1Fault)
  OR1/1 -> [B_SimComFaultA2]
  PULSE2/1 -> [B_SimComFaultA3], OR1/2, OR3/3
  B_TestLongTimeComFaultAllAxes/1 -> PULSE2/1
  ms2/1 -> PULSE2/2
  PULSE1/1 -> OR1/1, OR3/2
  B_TestLongTimeComFaultTwoAxes/1 -> PULSE1/1
  ms1/1 -> PULSE1/2
  PULSE/1 -> OR3/1
  OR3/1 -> [B_SimComFaultA1]
  ms/1 -> PULSE/2
  B_TestShortTimeComFault/1 -> PULSE/1
  AI_In_AEPAHeartbeatRecv1/1 -> USRB_Pitch_PitchCommunicationOK/1
  AI_In_AEPAHeartbeatRecv2/1 -> USRB_Pitch_PitchCommunicationOK1/1
  AI_In_AEPAHeartbeatRecv3/1 -> USRB_Pitch_PitchCommunicationOK2/1

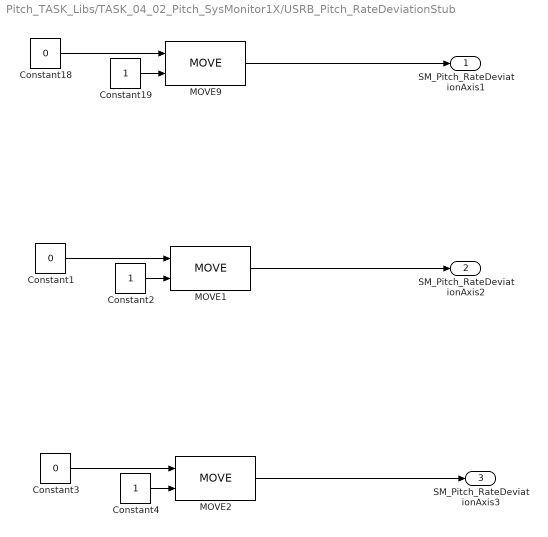
== system Pitch_TASK_Libs/TASK_04_02_Pitch_SysMonitor1X/USRB_Pitch_RateDeviationStub ==
  Constant1 : Constant  Value=0  OutDataTypeStr=boolean
  Constant18 : Constant  Value=0  OutDataTypeStr=boolean
  Constant19 : Constant  OutDataTypeStr=boolean
  Constant2 : Constant  OutDataTypeStr=boolean
  Constant3 : Constant  Value=0  OutDataTypeStr=boolean
  Constant4 : Constant  OutDataTypeStr=boolean
  MOVE1 : StandardLib/Memory operations/MOVE  DataType=BOOLEAN  SampleTime=-1  ExecutionOrder=0
  MOVE2 : StandardLib/Memory operations/MOVE  DataType=BOOLEAN  SampleTime=-1  ExecutionOrder=0
  MOVE9 : StandardLib/Memory operations/MOVE  DataType=BOOLEAN  SampleTime=-1  ExecutionOrder=0
  SM_Pitch_RateDeviationAxis1 : Outport  OutDataTypeStr=boolean
  SM_Pitch_RateDeviationAxis2 : Outport  Port=2  OutDataTypeStr=boolean
  SM_Pitch_RateDeviationAxis3 : Outport  Port=3  OutDataTypeStr=boolean
  wires:
  Constant19/1 -> MOVE9/2
  Constant18/1 -> MOVE9/1
  MOVE9/1 -> SM_Pitch_RateDeviationAxis1/1
  Constant2/1 -> MOVE1/2
  Constant1/1 -> MOVE1/1
  MOVE1/1 -> SM_Pitch_RateDeviationAxis2/1
  Constant4/1 -> MOVE2/2
  Constant3/1 -> MOVE2/1
  MOVE2/1 -> SM_Pitch_RateDeviationAxis3/1

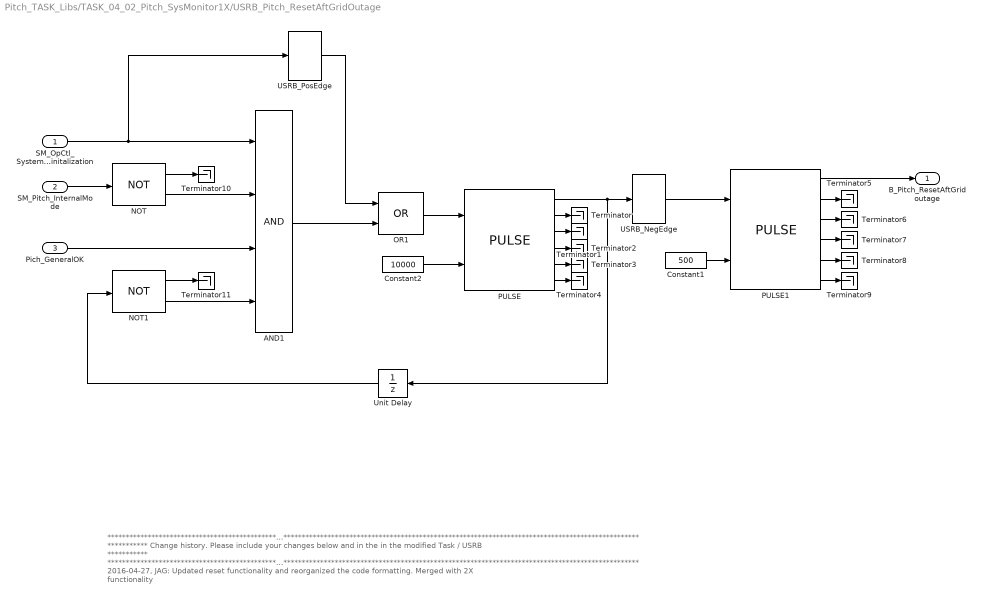
== system Pitch_TASK_Libs/TASK_04_02_Pitch_SysMonitor1X/USRB_Pitch_ResetAftGridOutage ==
  note: ***********************************************************************************************************************************************
      | ***********         Change history. Please include your changes below and in the in the modified Task / USRB         ***********
      | ***********************************************************************************************************************************************
      | 2016-04-27, JAG: Updated reset functionality and reorganized the code formatting. Merged with 2X functionality
  SM_OpCtl_SystemReinitalization : Inport  OutDataTypeStr=boolean
  SM_Pitch_InternalMode : Inport  Port=2  OutDataTypeStr=boolean
  Pich_GeneralOK : Inport  Port=3  OutDataTypeStr=boolean
  AND1 : StandardLib/Logical operations/AND  RepeatCnt=3  SampleTime=-1  ExecutionOrder=0
  Constant1 : Constant  Value=500  OutDataTypeStr=uint32
  Constant2 : Constant  Value=10000  OutDataTypeStr=uint32
  NOT : StandardLib/Logical operations/NOT  SampleTime=-1  ExecutionOrder=0
  NOT1 : StandardLib/Logical operations/NOT  SampleTime=-1  ExecutionOrder=0
  OR1 : StandardLib/Logical operations/OR  RepeatCnt=1  SampleTime=-1  ExecutionOrder=0
  PULSE : StandardLib/Sequencing/PULSE  SampleTime=-1  ExecutionOrder=0
  PULSE1 : StandardLib/Sequencing/PULSE  SampleTime=-1  ExecutionOrder=0
  Terminator{,1..11} (12 alike) : Terminator
  USRB_NegEdge : WindLib/USRB_NegEdge  SystemSampleTime=-1
  USRB_PosEdge : WindLib/USRB_PosEdge  SystemSampleTime=-1
  Unit Delay : UnitDelay  SampleTime=-1
  B_Pitch_ResetAftGridoutage : Outport  OutDataTypeStr=boolean
  wires:
  SM_OpCtl_SystemReinitalization/1 -> AND1/1, USRB_PosEdge/1
  PULSE/1 -> Unit Delay/1, USRB_NegEdge/1
  Pich_GeneralOK/1 -> AND1/3
  SM_Pitch_InternalMode/1 -> NOT/1
  NOT/2 -> AND1/2
  OR1/1 -> PULSE/1
  USRB_PosEdge/1 -> OR1/1
  AND1/1 -> OR1/2
  USRB_NegEdge/1 -> PULSE1/1
  Constant1/1 -> PULSE1/2
  PULSE1/1 -> B_Pitch_ResetAftGridoutage/1
  PULSE/2 -> Terminator/1
  PULSE/3 -> Terminator1/1
  PULSE/4 -> Terminator2/1
  PULSE/5 -> Terminator3/1
  PULSE/6 -> Terminator4/1
  PULSE1/2 -> Terminator5/1
  PULSE1/3 -> Terminator6/1
  PULSE1/4 -> Terminator7/1
  PULSE1/5 -> Terminator8/1
  PULSE1/6 -> Terminator9/1
  Constant2/1 -> PULSE/2
  NOT/1 -> Terminator10/1
  NOT1/1 -> Terminator11/1
  NOT1/2 -> AND1/4
  Unit Delay/1 -> NOT1/1

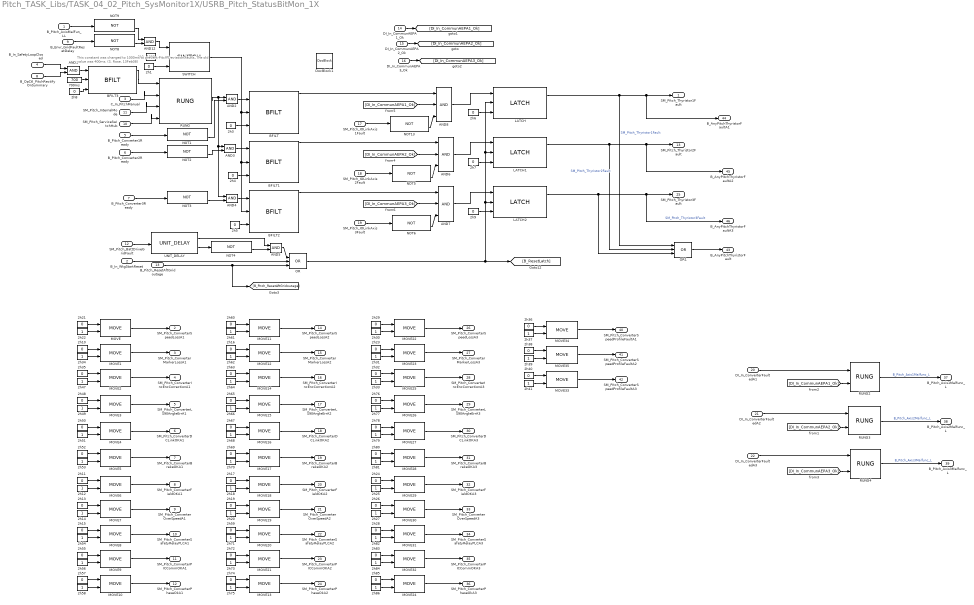
== system Pitch_TASK_Libs/TASK_04_02_Pitch_SysMonitor1X/USRB_Pitch_StatusBitMon_1X ==
  note: This constant was changed to 1000ms to prevent Pitch Deviation faults.
      | The old value was 400ms. (S. Rose, 13Feb08)
  B_Pitch_AxisMalFun_LL : Inport  OutDataTypeStr=boolean
  B_In_WtgStartReset : Inport  Port=2  OutDataTypeStr=boolean
  C_In_PitchManual : Inport  Port=3  OutDataTypeStr=boolean
  B_In_SafetyLoopClosed : Inport  Port=4  OutDataTypeStr=boolean
  B_Pitch_Converter1Ready : Inport  Port=5  OutDataTypeStr=boolean
  B_Pitch_Converter2Ready : Inport  Port=6  OutDataTypeStr=boolean
  B_Pitch_Converter3Ready : Inport  Port=7  OutDataTypeStr=boolean
  B_OpCtl_PitchRectifyOnSummary : Inport  Port=8  OutDataTypeStr=boolean
  B_Envr_GridFaultResetDelay : Inport  Port=9  OutDataTypeStr=boolean
  SM_Pitch_ServiceSwitchHub : Inport  Port=10  OutDataTypeStr=boolean
  SM_Pitch_InternalMode : Inport  Port=11  OutDataTypeStr=boolean
  SM_Pitch_BattDriveGridFault : Inport  Port=12  OutDataTypeStr=boolean
  B_Pitch_ResetAftGridoutage : Inport  Port=13  OutDataTypeStr=boolean
  DI_In_CommunAEPA1_Ok : Inport  Port=14  OutDataTypeStr=boolean
  DI_In_CommunAEPA2_Ok : Inport  Port=15  OutDataTypeStr=boolean
  DI_In_CommunAEPA3_Ok : Inport  Port=16  OutDataTypeStr=boolean
  SM_Pitch_IOLinkAxis1Fault : Inport  Port=17  OutDataTypeStr=boolean
  SM_Pitch_IOLinkAxis2Fault : Inport  Port=18  OutDataTypeStr=boolean
  SM_Pitch_IOLinkAxis3Fault : Inport  Port=19  OutDataTypeStr=boolean
  DI_In_ConverterFaultedA1 : Inport  Port=20  OutDataTypeStr=boolean
  DI_In_ConverterFaultedA2 : Inport  Port=21  OutDataTypeStr=boolean
  DI_In_ConverterFaultedA3 : Inport  Port=22  OutDataTypeStr=boolean
  2h{1,3..5,8} (5 alike) : Constant  Value=0  OutDataTypeStr=uint32
  2h{6..7,9..11,13,15..17,19,21,23..24,26,28..29,32,35..36,38,40,48,50,52,55,57,59..60,63,65,67,69,72,74,76,78,80,83,85} (39 alike) : Constant  Value=0  OutDataTypeStr=boolean
  2h{12,14,18,20,22,25,27,30..31,33..34,37,39,41,47,49,51,53..54,56,58,61..62,64,66,68,70..71,73,75,77,79,81..82,84,86} (36 alike) : Constant  OutDataTypeStr=boolean
  2h2 : Constant  Value=1000  OutDataTypeStr=uint32
  700ms : Constant  Value=700  OutDataTypeStr=uint32
  AND{1..5,12} (6 alike) : StandardLib/Logical operations/AND  RepeatCnt=1  SampleTime=-1  ExecutionOrder=0
  AND6 : StandardLib/Logical operations/AND  RepeatCnt=2  SampleTime=-1  ExecutionOrder=0
  AND7 : StandardLib/Logical operations/AND  RepeatCnt=2  SampleTime=-1  ExecutionOrder=0
  AND8 : StandardLib/Logical operations/AND  RepeatCnt=2  SampleTime=-1  ExecutionOrder=0
  BFILT{,1..3} (4 alike) : StandardLib/Filters/BFILT  SampleTime=-1  ExecutionOrder=0
  DocBlock1 : simulink/Model-Wide Utilities/DocBlock  SystemSampleTime=-1  DocumentType=Text
  LATCH : StandardLib/Logical operations/LATCH  SampleTime=-1  ExecutionOrder=0
  LATCH1 : StandardLib/Logical operations/LATCH  SampleTime=-1  ExecutionOrder=0
  LATCH2 : StandardLib/Logical operations/LATCH  SampleTime=-1  ExecutionOrder=0
  MOVE{,1..35} (36 alike) : StandardLib/Memory operations/MOVE  DataType=BOOLEAN  SampleTime=-1  ExecutionOrder=0
  NOT{1..6,8..9,13} (9 alike) : StandardLib/Logical operations/NOT  SampleTime=-1  ExecutionOrder=0
  OR : StandardLib/Logical operations/OR  RepeatCnt=2  SampleTime=-1  ExecutionOrder=0
  OR1 : StandardLib/Logical operations/OR  RepeatCnt=2  SampleTime=-1  ExecutionOrder=0
  RUNG : StandardLib/Logical operations/RUNG  Equation=(A*(~B)*(~C)*(~D))  RepeatCount=4  SampleTime=-1  ExecutionOrder=0
  RUNG2 : StandardLib/Logical operations/RUNG  Equation=A+~B  RepeatCount=2  SampleTime=-1  ExecutionOrder=0
  RUNG3 : StandardLib/Logical operations/RUNG  Equation=A+~B  RepeatCount=2  SampleTime=-1  ExecutionOrder=0
  RUNG4 : StandardLib/Logical operations/RUNG  Equation=A+~B  RepeatCount=2  SampleTime=-1  ExecutionOrder=0
  SWITCH : StandardLib/Memory operations/SWITCH  DataType=UINT32  SampleTime=-1  ExecutionOrder=0
  UNIT_DELAY : StandardLib/Memory operations/UNIT_DELAY  DataType=BOOLEAN  SampleTime=-1  ExecutionOrder=0
  SM_Pitch_Thyristor1Fault : Outport  OutDataTypeStr=boolean
  SM_Pitch_ConverterSpeedLossA1 : Outport  Port=2  OutDataTypeStr=boolean
  SM_Pitch_ConverterMarkerLossA1 : Outport  Port=3  OutDataTypeStr=boolean
  SM_Pitch_ConverterIncEncCorrectionA1 : Outport  Port=4  OutDataTypeStr=boolean
  SM_Pitch_ConverterLS90AngleErrA1 : Outport  Port=5  OutDataTypeStr=boolean
  SM_Pitch_ConverterDCLinkOKA1 : Outport  Port=6  OutDataTypeStr=boolean
  SM_Pitch_ConverterBrakeOKA1 : Outport  Port=7  OutDataTypeStr=boolean
  SM_Pitch_ConverterFieldOKA1 : Outport  Port=8  OutDataTypeStr=boolean
  SM_Pitch_ConverterOverSpeedA1 : Outport  Port=9  OutDataTypeStr=boolean
  SM_Pitch_ConverterSafetyRelayPLCA1 : Outport  Port=10  OutDataTypeStr=boolean
  SM_Pitch_ConverterPICCommOKA1 : Outport  Port=11  OutDataTypeStr=boolean
  SM_Pitch_ConverterPhaseOkA1 : Outport  Port=12  OutDataTypeStr=boolean
  SM_Pitch_Thyristor2Fault : Outport  Port=13  OutDataTypeStr=boolean
  SM_Pitch_ConverterSpeedLossA2 : Outport  Port=14  OutDataTypeStr=boolean
  SM_Pitch_ConverterMarkerLossA2 : Outport  Port=15  OutDataTypeStr=boolean
  SM_Pitch_ConverterIncEncCorrectionA2 : Outport  Port=16  OutDataTypeStr=boolean
  SM_Pitch_ConverterLS90AngleErrA2 : Outport  Port=17  OutDataTypeStr=boolean
  SM_Pitch_ConverterDCLinkOKA2 : Outport  Port=18  OutDataTypeStr=boolean
  SM_Pitch_ConverterBrakeOKA2 : Outport  Port=19  OutDataTypeStr=boolean
  SM_Pitch_ConverterFieldOKA2 : Outport  Port=20  OutDataTypeStr=boolean
  SM_Pitch_ConverterOverSpeedA2 : Outport  Port=21  OutDataTypeStr=boolean
  SM_Pitch_ConverterSafetyRelayPLCA2 : Outport  Port=22  OutDataTypeStr=boolean
  SM_Pitch_ConverterPICCommOKA2 : Outport  Port=23  OutDataTypeStr=boolean
  SM_Pitch_ConverterPhaseOkA2 : Outport  Port=24  OutDataTypeStr=boolean
  SM_Pitch_Thyristor3Fault : Outport  Port=25  OutDataTypeStr=boolean
  SM_Pitch_ConverterSpeedLossA3 : Outport  Port=26  OutDataTypeStr=boolean
  SM_Pitch_ConverterMarkerLossA3 : Outport  Port=27  OutDataTypeStr=boolean
  SM_Pitch_ConverterIncEncCorrectionA3 : Outport  Port=28  OutDataTypeStr=boolean
  SM_Pitch_ConverterLS90AngleErrA3 : Outport  Port=29  OutDataTypeStr=boolean
  SM_Pitch_ConverterDCLinkOKA3 : Outport  Port=30  OutDataTypeStr=boolean
  SM_Pitch_ConverterBrakeOKA3 : Outport  Port=31  OutDataTypeStr=boolean
  SM_Pitch_ConverterFieldOKA3 : Outport  Port=32  OutDataTypeStr=boolean
  SM_Pitch_ConverterOverSpeedA3 : Outport  Port=33  OutDataTypeStr=boolean
  SM_Pitch_ConverterSafetyRelayPLCA3 : Outport  Port=34  OutDataTypeStr=boolean
  SM_Pitch_ConverterPICCommOKA3 : Outport  Port=35  OutDataTypeStr=boolean
  SM_Pitch_ConverterPhaseOkA3 : Outport  Port=36  OutDataTypeStr=boolean
  B_Pitch_Axis1Malfunc_L : Outport  Port=37  OutDataTypeStr=boolean
  B_Pitch_Axis2Malfunc_L : Outport  Port=38  OutDataTypeStr=boolean
  B_Pitch_Axis3Malfunc_L : Outport  Port=39  OutDataTypeStr=boolean
  SM_Pitch_ConverterSpeedProfileFaultA1 : Outport  Port=40  OutDataTypeStr=boolean
  SM_Pitch_ConverterSpeedProfileFaultA2 : Outport  Port=41  OutDataTypeStr=boolean
  SM_Pitch_ConverterSpeedProfileFaultA3 : Outport  Port=42  OutDataTypeStr=boolean
  B_AnyPitchThyristorFault : Outport  Port=43  OutDataTypeStr=boolean
  B_AnyPitchThyristorFaultA1 : Outport  Port=44  OutDataTypeStr=boolean
  B_AnyPitchThyristorFaultA2 : Outport  Port=45  OutDataTypeStr=boolean
  B_AnyPitchThyristorFaultA3 : Outport  Port=46  OutDataTypeStr=boolean
  wires:
  B_Pitch_ResetAftGridoutage/1 -> OR/3, [B_Pitch_ResetAftGridoutage]
  LATCH2/1 -> OR1/3, SM_Pitch_Thyristor3Fault/1, B_AnyPitchThyristorFaultA3/1  "SM_Pitch_Thyristor3Fault"
  LATCH1/1 -> OR1/2, SM_Pitch_Thyristor2Fault/1, B_AnyPitchThyristorFaultA2/1  "SM_Pitch_Thyristor2Fault"
  B_In_SafetyLoopClosed/1 -> AND1/1
  B_OpCtl_PitchRectifyOnSummary/1 -> AND1/2
  AND1/1 -> BFILT3/1
  700ms/1 -> BFILT3/2
  2h8/1 -> BFILT3/3
  BFILT3/1 -> RUNG/1
  C_In_PitchManual/1 -> RUNG/2
  SM_Pitch_InternalMode/1 -> RUNG/3
  SM_Pitch_ServiceSwitchHub/1 -> RUNG/4
  B_Envr_GridFaultResetDelay/1 -> NOT8/1
  NOT8/2 -> AND12/2
  NOT9/2 -> AND12/1
  AND12/1 -> SWITCH/1
  2h2/1 -> SWITCH/2
  2h1/1 -> SWITCH/3
  B_Pitch_AxisMalFun_LL/1 -> NOT9/1
  B_Pitch_Converter1Ready/1 -> NOT1/1
  RUNG/1 -> AND2/1, AND3/1, AND4/1
  AND2/1 -> BFILT/1
  SWITCH/1 -> BFILT/2, BFILT1/2, BFILT2/2
  2h3/1 -> BFILT/3
  B_Pitch_Converter2Ready/1 -> NOT2/1
  2h4/1 -> BFILT1/3
  NOT1/2 -> AND2/2
  NOT2/2 -> AND3/2
  AND3/1 -> BFILT1/1
  2h5/1 -> BFILT2/3
  AND4/1 -> BFILT2/1
  B_Pitch_Converter3Ready/1 -> NOT3/1
  NOT3/2 -> AND4/2
  B_In_WtgStartReset/1 -> OR/2
  SM_Pitch_BattDriveGridFault/1 -> UNIT_DELAY/1
  UNIT_DELAY/2 -> NOT4/1
  UNIT_DELAY/1 -> AND5/1
  NOT4/2 -> AND5/2
  AND5/1 -> OR/1
  2h6/1 -> LATCH/3
  2h7/1 -> LATCH1/3
  2h9/1 -> LATCH2/3
  OR/1 -> LATCH/2, LATCH1/2, LATCH2/2, [B_ResetLatch]
  LATCH/1 -> OR1/1, SM_Pitch_Thyristor1Fault/1, B_AnyPitchThyristorFaultA1/1  "SM_Pitch_Thyristor1Fault"
  NOT13/2 -> AND8/3
  SM_Pitch_IOLinkAxis1Fault/1 -> NOT13/1
  BFILT/1 -> AND8/1
  AND8/1 -> LATCH/1
  NOT5/2 -> AND6/3
  SM_Pitch_IOLinkAxis2Fault/1 -> NOT5/1
  BFILT1/1 -> AND6/1
  AND6/1 -> LATCH1/1
  NOT6/2 -> AND7/3
  SM_Pitch_IOLinkAxis3Fault/1 -> NOT6/1
  BFILT2/1 -> AND7/1
  AND7/1 -> LATCH2/1
  [DI_In_CommunAEPA1_Ok] -> RUNG2/2
  RUNG3/1 -> B_Pitch_Axis2Malfunc_L/1  "B_Pitch_Axis2Malfunc_L"
  DI_In_ConverterFaultedA3/1 -> RUNG4/1
  RUNG4/1 -> B_Pitch_Axis3Malfunc_L/1  "B_Pitch_Axis3Malfunc_L"
  DI_In_ConverterFaultedA2/1 -> RUNG3/1
  RUNG2/1 -> B_Pitch_Axis1Malfunc_L/1  "B_Pitch_Axis1Malfunc_L"
  DI_In_ConverterFaultedA1/1 -> RUNG2/1
  DI_In_CommunAEPA2_Ok/1 -> [DI_In_CommunAEPA2_Ok]
  DI_In_CommunAEPA1_Ok/1 -> [DI_In_CommunAEPA1_Ok]
  DI_In_CommunAEPA3_Ok/1 -> [DI_In_CommunAEPA3_Ok]
  [DI_In_CommunAEPA2_Ok] -> RUNG3/2
  [DI_In_CommunAEPA3_Ok] -> RUNG4/2
  [DI_In_CommunAEPA1_Ok] -> AND8/2
  [DI_In_CommunAEPA2_Ok] -> AND6/2
  [DI_In_CommunAEPA3_Ok] -> AND7/2
  OR1/1 -> B_AnyPitchThyristorFault/1
  2h21/1 -> MOVE/1
  2h22/1 -> MOVE/2
  MOVE/1 -> SM_Pitch_ConverterSpeedLossA1/1
  2h10/1 -> MOVE1/1
  2h34/1 -> MOVE1/2
  2h35/1 -> MOVE2/1
  2h47/1 -> MOVE2/2
  2h48/1 -> MOVE3/1
  2h49/1 -> MOVE3/2
  2h50/1 -> MOVE4/1
  2h51/1 -> MOVE4/2
  2h52/1 -> MOVE5/1
  2h53/1 -> MOVE5/2
  MOVE1/1 -> SM_Pitch_ConverterMarkerLossA1/1
  MOVE2/1 -> SM_Pitch_ConverterIncEncCorrectionA1/1
  MOVE3/1 -> SM_Pitch_ConverterLS90AngleErrA1/1
  MOVE4/1 -> SM_Pitch_ConverterDCLinkOKA1/1
  2h11/1 -> MOVE6/1
  2h12/1 -> MOVE6/2
  2h13/1 -> MOVE7/1
  2h14/1 -> MOVE7/2
  2h15/1 -> MOVE8/1
  2h54/1 -> MOVE8/2
  2h55/1 -> MOVE9/1
  2h56/1 -> MOVE9/2
  2h57/1 -> MOVE10/1
  2h58/1 -> MOVE10/2
  MOVE10/1 -> SM_Pitch_ConverterPhaseOkA1/1
  MOVE9/1 -> SM_Pitch_ConverterPICCommOKA1/1
  MOVE8/1 -> SM_Pitch_ConverterSafetyRelayPLCA1/1
  MOVE7/1 -> SM_Pitch_ConverterOverSpeedA1/1
  MOVE6/1 -> SM_Pitch_ConverterFieldOKA1/1
  MOVE5/1 -> SM_Pitch_ConverterBrakeOKA1/1
  2h60/1 -> MOVE11/1
  2h61/1 -> MOVE11/2
  2h16/1 -> MOVE12/1
  2h62/1 -> MOVE12/2
  2h63/1 -> MOVE14/1
  2h64/1 -> MOVE14/2
  2h65/1 -> MOVE15/1
  2h66/1 -> MOVE15/2
  2h67/1 -> MOVE16/1
  2h68/1 -> MOVE16/2
  2h69/1 -> MOVE17/1
  2h70/1 -> MOVE17/2
  2h17/1 -> MOVE18/1
  2h18/1 -> MOVE18/2
  2h19/1 -> MOVE19/1
  2h20/1 -> MOVE19/2
  2h59/1 -> MOVE20/1
  2h71/1 -> MOVE20/2
  2h72/1 -> MOVE21/1
  2h73/1 -> MOVE21/2
  2h74/1 -> MOVE13/1
  2h75/1 -> MOVE13/2
  MOVE11/1 -> SM_Pitch_ConverterSpeedLossA2/1
  MOVE12/1 -> SM_Pitch_ConverterMarkerLossA2/1
  MOVE14/1 -> SM_Pitch_ConverterIncEncCorrectionA2/1
  MOVE15/1 -> SM_Pitch_ConverterLS90AngleErrA2/1
  MOVE16/1 -> SM_Pitch_ConverterDCLinkOKA2/1
  MOVE17/1 -> SM_Pitch_ConverterBrakeOKA2/1
  MOVE18/1 -> SM_Pitch_ConverterFieldOKA2/1
  MOVE19/1 -> SM_Pitch_ConverterOverSpeedA2/1
  MOVE21/1 -> SM_Pitch_ConverterPICCommOKA2/1
  MOVE13/1 -> SM_Pitch_ConverterPhaseOkA2/1
  MOVE20/1 -> SM_Pitch_ConverterSafetyRelayPLCA2/1
  2h29/1 -> MOVE22/1
  2h30/1 -> MOVE22/2
  2h23/1 -> MOVE23/1
  2h31/1 -> MOVE23/2
  2h32/1 -> MOVE25/1
  2h33/1 -> MOVE25/2
  2h76/1 -> MOVE26/1
  2h77/1 -> MOVE26/2
  2h78/1 -> MOVE27/1
  2h79/1 -> MOVE27/2
  2h80/1 -> MOVE28/1
  2h81/1 -> MOVE28/2
  2h24/1 -> MOVE29/1
  2h25/1 -> MOVE29/2
  2h26/1 -> MOVE30/1
  2h27/1 -> MOVE30/2
  2h28/1 -> MOVE31/1
  2h82/1 -> MOVE31/2
  2h83/1 -> MOVE32/1
  2h84/1 -> MOVE32/2
  2h85/1 -> MOVE24/1
  2h86/1 -> MOVE24/2
  MOVE22/1 -> SM_Pitch_ConverterSpeedLossA3/1
  MOVE23/1 -> SM_Pitch_ConverterMarkerLossA3/1
  MOVE25/1 -> SM_Pitch_ConverterIncEncCorrectionA3/1
  MOVE26/1 -> SM_Pitch_ConverterLS90AngleErrA3/1
  MOVE27/1 -> SM_Pitch_ConverterDCLinkOKA3/1
  MOVE28/1 -> SM_Pitch_ConverterBrakeOKA3/1
  MOVE29/1 -> SM_Pitch_ConverterFieldOKA3/1
  MOVE30/1 -> SM_Pitch_ConverterOverSpeedA3/1
  MOVE24/1 -> SM_Pitch_ConverterPhaseOkA3/1
  MOVE32/1 -> SM_Pitch_ConverterPICCommOKA3/1
  MOVE31/1 -> SM_Pitch_ConverterSafetyRelayPLCA3/1
  2h36/1 -> MOVE34/1
  2h37/1 -> MOVE34/2
  2h38/1 -> MOVE35/1
  2h39/1 -> MOVE35/2
  2h40/1 -> MOVE33/1
  2h41/1 -> MOVE33/2
  MOVE33/1 -> SM_Pitch_ConverterSpeedProfileFaultA3/1
  MOVE35/1 -> SM_Pitch_ConverterSpeedProfileFaultA2/1
  MOVE34/1 -> SM_Pitch_ConverterSpeedProfileFaultA1/1
